simulink model "divergence_sim2"  (R2025b)
settings: Solver=VariableStepAuto  StartTime=0.0  StopTime=3  RelTol=1e-3
PreLoadFcn:
  | % PreLoadFcn - 最小構成
  | stlFile = fullfile(pwd, 'mazeActor.stl');
  | assignin('base', 'stlFile', stlFile);
InitFcn:
  | inputImage = fullfile(pwd, '', 'ex_maze.png');
  | assignin('base', 'mazeInputImage', inputImage);
  | 
  | % InitFcn - 最小構成
  | % Base ワークスペースから変数を取得（無ければエラー）
  | if ~evalin('base','exist(''mazeInputImage'',''var'')')
  |     error('InitFcn:NoInputVar','mazeInputImage not found in base workspace. Ensure PreLoadFcn ran.');
  | end
  | if ~evalin('base','exist(''stlFile'',''var'')')
  |     error('InitFcn:NoSTLVar','stlFile not found in base workspace. Ensure PreLoadFcn ran.');
  | end
  | 
  | inputImage = evalin('base','mazeInputImage');
  | stlFile    = evalin('base','stlFile');
  | 
  | % 入力確認（最小チェック）
  | if ~isfile(inputImage)
  |     error('InitFcn:NoInputFile','Input image not found: %s', inputImage);
  | end
  | 
  | % 実処理：STL 生成（prepareMazeSTL は既存関数と仮定）
  | prepareMazeSTL(inputImage);
  | 
  | % (必要なら prepareMazeSTL 内で stlFile を参照するか、関数に渡す設計にする)
undefined symbols (not defined in the file or in its folder): DiscIntNeverNeededParam, Sim3dSensor
libraries: sim3dlib x3, sim3dgroundtruthsensorlib x3
settings Model: Creator=akina  LastModifiedBy=akina
settings SFSimCC: SimUserSources=cfolder/solver.c  SFSimEcho=off

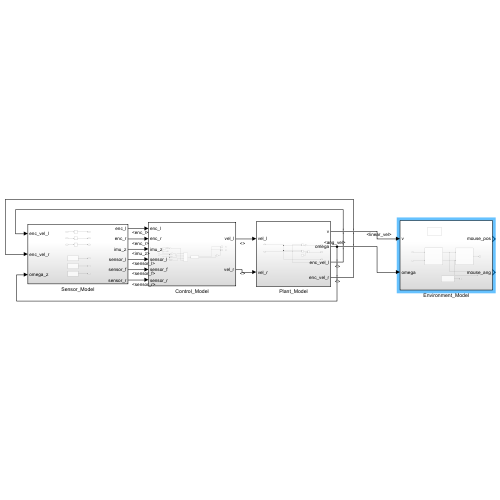
[thumbnail: Simulink's stored preview of the top-level diagram]
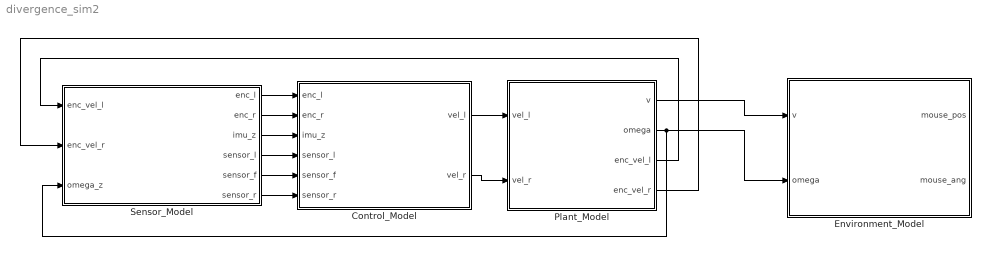
== system divergence_sim2 ==
  Control_Model : Subsystem
  Environment_Model : Subsystem
  Plant_Model : Subsystem
  Sensor_Model : Subsystem
  wires:
  Plant_Model/1(v) -> Environment_Model/1(v)
  Control_Model/1(vel_l) -> Plant_Model/1(vel_l)
  Control_Model/2(vel_r) -> Plant_Model/2(vel_r)
  Plant_Model/2(omega) -> Sensor_Model/3(omega_z), Environment_Model/2(omega)
  Sensor_Model/1(enc_l) -> Control_Model/1(enc_l)
  Sensor_Model/2(enc_r) -> Control_Model/2(enc_r)
  Plant_Model/3(enc_vel_l) -> Sensor_Model/1(enc_vel_l)
  Plant_Model/4(enc_vel_r) -> Sensor_Model/2(enc_vel_r)
  Sensor_Model/3(imu_z) -> Control_Model/3(imu_z)
  Sensor_Model/4(sensor_l) -> Control_Model/4(sensor_l)
  Sensor_Model/5(sensor_f) -> Control_Model/5(sensor_f)
  Sensor_Model/6(sensor_r) -> Control_Model/6(sensor_r)

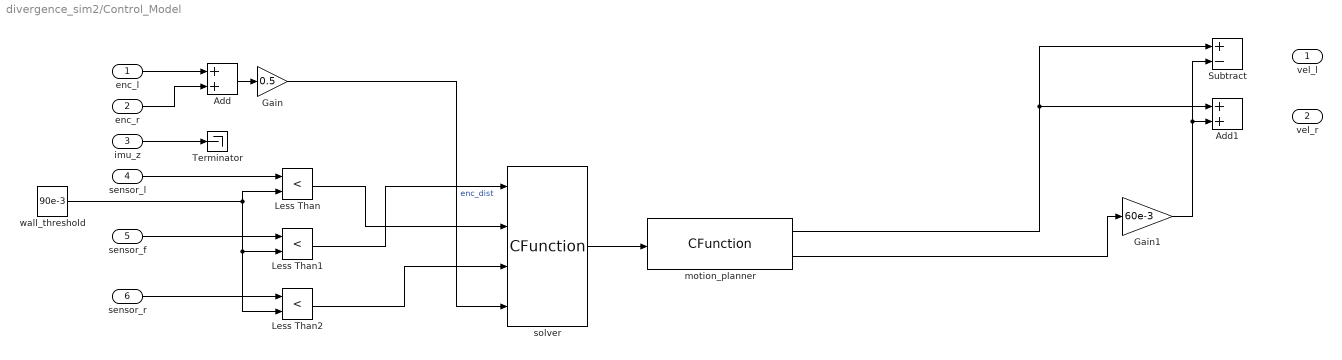
== system divergence_sim2/Control_Model ==
  enc_l : Inport
  enc_r : Inport  Port=2
  imu_z : Inport  Port=3
  sensor_l : Inport  Port=4
  sensor_f : Inport  Port=5
  sensor_r : Inport  Port=6
  Add : Sum
  Add1 : Sum
  Gain : Gain  Gain=0.5
  Gain1 : Gain  Gain=60e-3
  Less Than : RelationalOperator  Operator=<  OutDataTypeStr=boolean  RndMeth=Simplest  InputSameDT=off
  Less Than1 : RelationalOperator  Operator=<  OutDataTypeStr=boolean  RndMeth=Simplest  InputSameDT=off
  Less Than2 : RelationalOperator  Operator=<  OutDataTypeStr=boolean  RndMeth=Simplest  InputSameDT=off
  Subtract : Sum  Inputs=+-
  Terminator : Terminator
  motion_planner : CFunction  OutputCode=|  CodegenOutputCode=|
      OutputCode=|
      | typedef enum {
      |     STOP,
      |     FORWARD,
      |     TURN_LEFT,
      |     TURN_RIGHT,
      |     TURN_BACK
      | } MotionState;
      | 
      | void motion_planner(
      |     int action,
      |     double *v_ref,
      |     double *w_ref)
      | {
      |     static MotionState state = STOP;
      | 
      |     const double V = 0.3;
      |     const double W = 6.0;
      | 
      |     if(action != -1)
      |     {
      |         if(action == 0) state = FORWARD;
      |         if(action == 1) state = TURN_LEFT;
      |         if(action == 2) state = TURN_RIGHT;
      |         if(action == 3) state = TURN_BACK;
      |     }
      | 
      |     switch(state)
      |     {
      |         case FORWARD:
      |             *v_ref = V;
      |             *w_ref = 0;
      |             break;
      | 
      |         case TURN_LEFT:
      |             *v_ref = 0;
      |             *w_ref = W;
      |             break;
      | 
      |         case TURN_RIGHT:
      |             *v_ref = 0;
      |             *w_ref = -W;
      |             break;
      | 
      |         case TURN_BACK:
      |             *v_ref = 0;
      |             *w_ref = W;
      |             break;
      | 
      |         default:
      |             *v_ref = 0;
      |             *w_ref = 0;
      |     }
      | }
      CodegenOutputCode=|
      | typedef enum {
      |     STOP,
      |     FORWARD,
      |     TURN_LEFT,
      |     TURN_RIGHT,
      |     TURN_BACK
      | } MotionState;
      | 
      | void motion_planner(
      |     int action,
      |     double *v_ref,
      |     double *w_ref)
      | {
      |     static MotionState state = STOP;
      | 
      |     const double V = 0.3;
      |     const double W = 6.0;
      | 
      |     if(action != -1)
      |     {
      |         if(action == 0) state = FORWARD;
      |         if(action == 1) state = TURN_LEFT;
      |         if(action == 2) state = TURN_RIGHT;
      |         if(action == 3) state = TURN_BACK;
      |     }
      | 
      |     switch(state)
      |     {
      |         case FORWARD:
      |             *v_ref = V;
      |             *w_ref = 0;
      |             break;
      | 
      |         case TURN_LEFT:
      |             *v_ref = 0;
      |             *w_ref = W;
      |             break;
      | 
      |         case TURN_RIGHT:
      |             *v_ref = 0;
      |             *w_ref = -W;
      |             break;
      | 
      |         case TURN_BACK:
      |             *v_ref = 0;
      |             *w_ref = W;
      |             break;
      | 
      |         default:
      |             *v_ref = 0;
      |             *w_ref = 0;
      |     }
      | }
  solver : CFunction  OutputCode=|  CodegenOutputCode=|
      OutputCode=|
      | void solver(
      |     int front,
      |     int left,
      |     int right,
      |     double distance,
      |     int *action)
      | {
      | 
      |     const double CELL = 0.18;
      |     static double next_call = 0.18;
      | 
      |     *action = -1;
      |     if(distance >= next_cell)
      |     {
      |         if(!left) {
      |         *action = 1;
      |         } else if(!front) {
      |             *action = 0;
      |         } else if(!right) {
      |             *action = 2;
      |         } else {
      |             *action = 3;
      |         }
      |     }
      | }
      CodegenOutputCode=|
      | void solver(
      |     int front,
      |     int left,
      |     int right,
      |     double distance,
      |     int *action)
      | {
      | 
      |     const double CELL = 0.18;
      |     static double next_call = 0.18;
      | 
      |     *action = -1;
      |     if(distance >= next_cell)
      |     {
      |         if(!left) {
      |         *action = 1;
      |         } else if(!front) {
      |             *action = 0;
      |         } else if(!right) {
      |             *action = 2;
      |         } else {
      |             *action = 3;
      |         }
      |     }
      | }
  wall_threshold : Constant  Value=90e-3
  vel_l : Outport
  vel_r : Outport  Port=2
  wires:
  sensor_l/1 -> Less Than/1
  wall_threshold/1 -> Less Than/2, Less Than2/2, Less Than1/2
  sensor_f/1 -> Less Than1/1
  sensor_r/1 -> Less Than2/1
  enc_l/1 -> Add/1
  enc_r/1 -> Add/2
  Add/1 -> Gain/1
  imu_z/1 -> Terminator/1
  motion_planner/2 -> Gain1/1
  Gain1/1 -> Add1/2, Subtract/2
  motion_planner/1 -> Add1/1, Subtract/1
  Less Than/1 -> solver/2
  Less Than1/1 -> solver/1
  Less Than2/1 -> solver/3
  solver/1 -> motion_planner/1
  Gain/1 -> solver/4  "enc_dist"

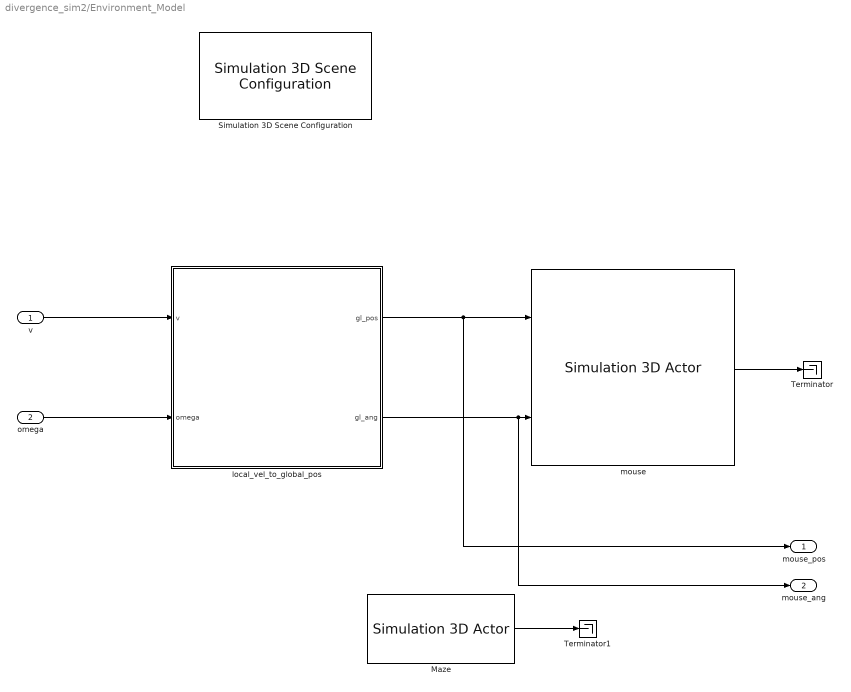
== system divergence_sim2/Environment_Model ==
  v : Inport
  omega : Inport  Port=2
  Maze : sim3dlib/Simulation 3D Actor  Priority=1  ActorName=Sim3dActor1  ParentName=Scene Origin  Operation=Create at setup  InitScriptText=|  SampleTime=-1  Translation=[-0.09 -2.88+0.09 0]  Rotation=[0 0 0]  Scale=[1 1 1]  aMode=5  ActorTag=Sim3dActor1  ActorType=Sim3dActor  ID=1
      | Actor.PreciseContacts = false;
      | Actor.Physics = false;
      | Actor.Color = [1 1 1];
      | actor.Shininess = 0;
      | actor.Metallic = 0;
      | Actor.Collisions = false;
  Simulation 3D Scene Configuration : sim3dlib/Simulation 3D Scene Configuration  Priority=0  ProjectFormat=Default Scenes  SceneDesc=Empty scene  ProjectName=C:\Program Files\MATLAB\R2025b\toolbox\shared\sim3d_projects\automotive_project_windows\UE\WindowsNoEditor\VehicleSimulation.exe  ScenePath=/Game/Maps/HwStrght  EnableOpenDRIVE=off  vehTagList={'Custom';'Scene Origin'}  vehTag=Custom  AttachedCameraRelativeTranslation=[0 0 0]  FreeCameraDefaultInitialTranslation=[-6, 0, 2]  AttachedCameraRelativeRotation=[0 0 0]  FreeCameraDefaultInitialRotation=[0, -15, 0]  ViewpointName=Custom  FreeCameraInitialTranslation=[0 0.6 1.5]  ViewpointTranslation=[0 0 0]  FreeCameraInitialRotation=[0 -90 -90]  ViewpointRotation=[0 0 0]  OpVisEn=off  Ts=.001  EnableWindow=on  EnableRemoteAccess=off  EnableWeather=off  SunAzimuth=90  SunAltitude=40.0  EnableGeospatialSun=off  Latitude=0  Longitude=0  Date=2023-01-01  Time=10:30:00  GeoTimeZone=-5.0  SunDaylightSaving=off  wind=1  clouds=10  EnableVolumetricClouds=off  CloudCoverage=0  CloudAltitude=6  fog=0  rain=0  RaindropsEffect=off  SnowDensity=0  EnableGeospatial=off  TilesetSource=Earth terrain  UseTrueOrigin=off  OriginHeight=200  OriginLatitude=40.744652  OriginLongitude=-73.988864  MapStyle=Aerial  AdditionalAssetIDs=[]  UseAdvancedSunSky=off  SolarTime=11  TimeZone=-5  Day=21  Month=9  Year=2022  UseDaylightSavingTime=on  DSTStartDay=10  DSTStartMonth=3  DSTEndDay=3  DSTEndMonth=11  DSTSwitchHour=2  sensorTag=MainCamera1  sensorId=1  sensorName=MainCamera1  mountLoc=Origin  offsetFlag=off  tmountOffset=[0, 0, 0]  rmountOffset=[0, 0, 0]  HorizontalResolution=1280  VerticalResolution=720  HorizontalFOV=60  mountPoint=[0 0 0]  mountOrientation=[0 0 0]  aMode=5  ID=1  GeoTrigger=Inactive  ViewNameList={'Custom'}  ViewTranslationList={'[0 0.6 1.5]'}  ViewRotationList={'[0 -90 -90]'}
      settings: LibrarySourceBlock=sl3dlib/Simulation 3D/Environment/Simulation 3D Scene Configuration
  Terminator : Terminator
  Terminator1 : Terminator
  local_vel_to_global_pos : Subsystem
  mouse : sim3dlib/Simulation 3D Actor  Priority=1  ActorName=Mouse  ParentName=Scene Origin  Operation=Create at setup  InitScriptText=|  SampleTime=-1  Translation=[0 0 0]  Rotation=[0 0 0]  Scale=[1 1 1]*1e-3  InputsText=Mouse.Translation Mouse.Rotation  aMode=5  ActorTag=Mouse  ActorType=Sim3dActor  ID=C
      | Actor.Shadows = false;
      | Actor.Collisions = false;
      | Actor.Color = [0,0,0];
  mouse_pos : Outport
  mouse_ang : Outport  Port=2
  wires:
  mouse/1 -> Terminator/1
  v/1 -> local_vel_to_global_pos/1(v)
  omega/1 -> local_vel_to_global_pos/2(omega)
  Maze/1 -> Terminator1/1
  local_vel_to_global_pos/1(gl_pos) -> mouse_pos/1, mouse/1
  local_vel_to_global_pos/2(gl_ang) -> mouse_ang/1, mouse/2

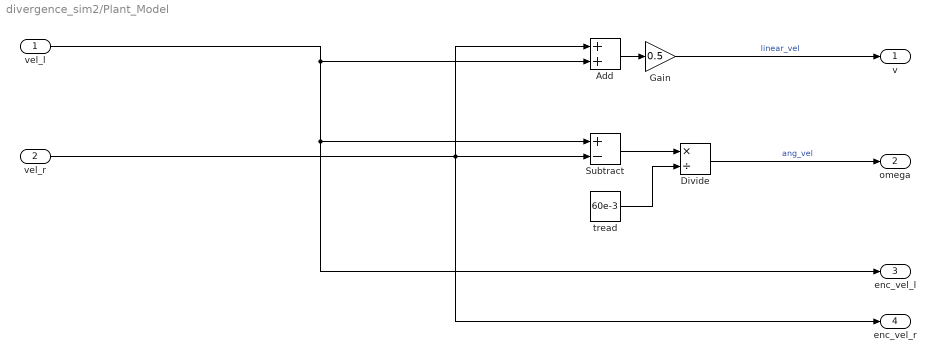
== system divergence_sim2/Plant_Model ==
  vel_l : Inport
  vel_r : Inport  Port=2
  Add : Sum
  Divide : Product  Inputs=*/
  Gain : Gain  Gain=0.5
  Subtract : Sum  Inputs=+-
  tread : Constant  Value=60e-3
  v : Outport
  omega : Outport  Port=2
  enc_vel_l : Outport  Port=3
  enc_vel_r : Outport  Port=4
  wires:
  Add/1 -> Gain/1
  Subtract/1 -> Divide/1
  Divide/1 -> omega/1  "ang_vel"
  tread/1 -> Divide/2
  Gain/1 -> v/1  "linear_vel"
  vel_l/1 -> enc_vel_l/1, Subtract/1, Add/2
  vel_r/1 -> enc_vel_r/1, Subtract/2, Add/1

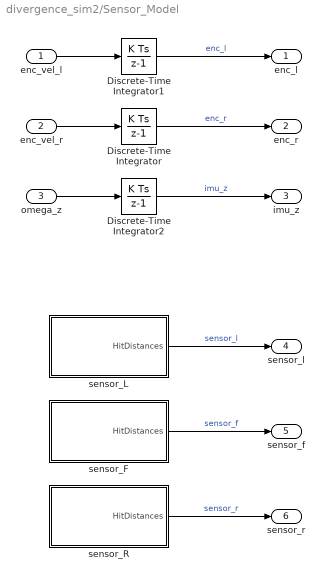
== system divergence_sim2/Sensor_Model ==
  enc_vel_l : Inport
  enc_vel_r : Inport  Port=2
  omega_z : Inport  Port=3
  Discrete-Time Integrator : DiscreteIntegrator  SampleTime=-1  ICPrevOutput=DiscIntNeverNeededParam  ICPrevScaledInput=DiscIntNeverNeededParam
  Discrete-Time Integrator1 : DiscreteIntegrator  SampleTime=-1  ICPrevOutput=DiscIntNeverNeededParam  ICPrevScaledInput=DiscIntNeverNeededParam
  Discrete-Time Integrator2 : DiscreteIntegrator  SampleTime=-1  ICPrevOutput=DiscIntNeverNeededParam  ICPrevScaledInput=DiscIntNeverNeededParam
  sensor_F : Subsystem  mask{pos_x=60, pos_y=0, ang_z=0}
      mask prompts: pos_x "sensor position x (mm)"; pos_y "sensor position y (mm)"; ang_z "sensor rotation z (deg)"
      mask DialogControl ParameterGroupVar Prompt: パラメーター
  sensor_L : Subsystem  mask{pos_x=60, pos_y=0, ang_z=-60}
      mask prompts: pos_x "sensor position x (mm)"; pos_y "sensor position y (mm)"; ang_z "sensor rotation z (deg)"
      mask DialogControl ParameterGroupVar Prompt: パラメーター
  sensor_R : Subsystem  mask{pos_x=60, pos_y=0, ang_z=60}
      mask prompts: pos_x "sensor position x (mm)"; pos_y "sensor position y (mm)"; ang_z "sensor rotation z (deg)"
      mask DialogControl ParameterGroupVar Prompt: パラメーター
  enc_l : Outport
  enc_r : Outport  Port=2
  imu_z : Outport  Port=3
  sensor_l : Outport  Port=4
  sensor_f : Outport  Port=5
  sensor_r : Outport  Port=6
  wires:
  enc_vel_r/1 -> Discrete-Time Integrator/1
  enc_vel_l/1 -> Discrete-Time Integrator1/1
  Discrete-Time Integrator/1 -> enc_r/1  "enc_r"
  Discrete-Time Integrator1/1 -> enc_l/1  "enc_l"
  omega_z/1 -> Discrete-Time Integrator2/1
  Discrete-Time Integrator2/1 -> imu_z/1  "imu_z"
  sensor_F/1(HitDistances) -> sensor_f/1  "sensor_f"
  sensor_R/1(HitDistances) -> sensor_r/1  "sensor_r"
  sensor_L/1(HitDistances) -> sensor_l/1  "sensor_l"

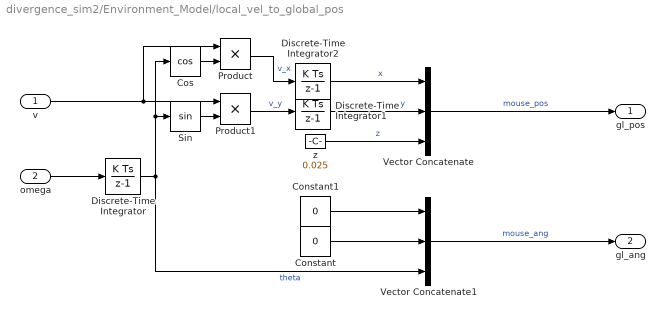
== system divergence_sim2/Environment_Model/local_vel_to_global_pos ==
  v : Inport
  omega : Inport  Port=2
  Constant : Constant  Value=0
  Constant1 : Constant  Value=0
  Cos : Trigonometry  Operator=cos
  Discrete-Time Integrator : DiscreteIntegrator  InitialCondition=-pi/2  SampleTime=-1  ICPrevOutput=DiscIntNeverNeededParam  ICPrevScaledInput=DiscIntNeverNeededParam
  Discrete-Time Integrator1 : DiscreteIntegrator  SampleTime=-1  ICPrevOutput=DiscIntNeverNeededParam  ICPrevScaledInput=DiscIntNeverNeededParam
  Discrete-Time Integrator2 : DiscreteIntegrator  SampleTime=-1  ICPrevOutput=DiscIntNeverNeededParam  ICPrevScaledInput=DiscIntNeverNeededParam
  Product : Product
  Product1 : Product
  Sin : Trigonometry
  Vector Concatenate : Concatenate  NumInputs=3  Mode=Multidimensional array  ConcatenateDimension=2
  Vector Concatenate1 : Concatenate  NumInputs=3  Mode=Multidimensional array  ConcatenateDimension=2
  z : Constant  Value=0.025
  gl_pos : Outport
  gl_ang : Outport  Port=2
  wires:
  omega/1 -> Discrete-Time Integrator/1
  Discrete-Time Integrator/1 -> Vector Concatenate1/3, Sin/1, Cos/1  "theta"
  Product1/1 -> Discrete-Time Integrator1/1  "v_y"
  Product/1 -> Discrete-Time Integrator2/1  "v_x"
  v/1 -> Product1/1, Product/1
  Cos/1 -> Product/2
  Sin/1 -> Product1/2
  Discrete-Time Integrator2/1 -> Vector Concatenate/1  "x"
  Discrete-Time Integrator1/1 -> Vector Concatenate/2  "y"
  z/1 -> Vector Concatenate/3  "z"
  Constant1/1 -> Vector Concatenate1/1
  Constant/1 -> Vector Concatenate1/2
  Vector Concatenate/1 -> gl_pos/1  "mouse_pos"
  Vector Concatenate1/1 -> gl_ang/1  "mouse_ang"

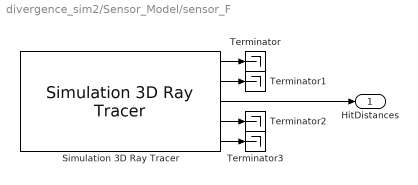
== system divergence_sim2/Sensor_Model/sensor_F ==
  Simulation 3D Ray Tracer : sim3dgroundtruthsensorlib/Simulation 3D Ray Tracer  Priority=1  sensorTag=Sim3dSensor�  sensorId=1  sensorName=Sim3dSensor�  vehTagList={'Mouse';'Scene Origin';'Sim3dActor1'}  vehTag=Mouse  CoordinateSystem=Default  mountLoc=Origin  offsetFlag=on  tmountOffset=[pos_x pos_y 2]  rmountOffset=[0 -pi/2 ang_z/180*pi]  RayOrigins=[0 0 0]  RayDirections=[0 0 1]  RayLengths=4000  NumberOfBounces=0  VisualizeTraceLines=on  EnableOptimization=off  SampleTime=-1  mountPoint=[60 0 2]  mountOrientation=[0 -1.5707963267949 0]  aMode=5  ID=1
      settings: LibrarySourceBlock=sl3dlib/Simulation 3D/Sensors/Simulation 3D Ray Tracer
  Terminator{,1..3} (4 alike) : Terminator
  HitDistances : Outport
  wires:
  Simulation 3D Ray Tracer/3 -> HitDistances/1
  Simulation 3D Ray Tracer/2 -> Terminator1/1
  Simulation 3D Ray Tracer/4 -> Terminator2/1
  Simulation 3D Ray Tracer/5 -> Terminator3/1
  Simulation 3D Ray Tracer/1 -> Terminator/1

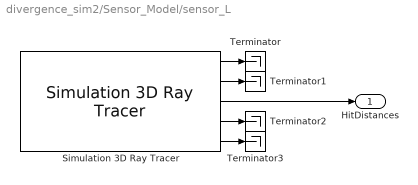
== system divergence_sim2/Sensor_Model/sensor_L ==
  Simulation 3D Ray Tracer : sim3dgroundtruthsensorlib/Simulation 3D Ray Tracer  Priority=1  sensorTag=Sim3dSensor�  sensorId=3  sensorName=Sim3dSensor�  vehTagList={'Mouse';'Scene Origin';'Sim3dActor1'}  vehTag=Mouse  CoordinateSystem=Default  mountLoc=Origin  offsetFlag=on  tmountOffset=[pos_x pos_y 2]  rmountOffset=[0 -pi/2 ang_z/180*pi]  RayOrigins=[0 0 0]  RayDirections=[0 0 1]  RayLengths=4000  NumberOfBounces=0  VisualizeTraceLines=on  EnableOptimization=off  SampleTime=-1  mountPoint=[60 0 2]  mountOrientation=[0 -1.5707963267949 -1.0471975511966]  aMode=5  ID=3
      settings: LibrarySourceBlock=sl3dlib/Simulation 3D/Sensors/Simulation 3D Ray Tracer
  Terminator{,1..3} (4 alike) : Terminator
  HitDistances : Outport
  wires:
  Simulation 3D Ray Tracer/3 -> HitDistances/1
  Simulation 3D Ray Tracer/2 -> Terminator1/1
  Simulation 3D Ray Tracer/4 -> Terminator2/1
  Simulation 3D Ray Tracer/5 -> Terminator3/1
  Simulation 3D Ray Tracer/1 -> Terminator/1

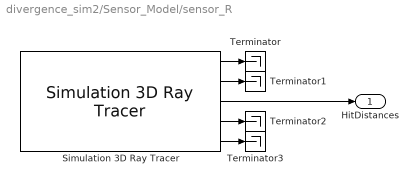
== system divergence_sim2/Sensor_Model/sensor_R ==
  Simulation 3D Ray Tracer : sim3dgroundtruthsensorlib/Simulation 3D Ray Tracer  Priority=1  sensorTag=Sim3dSensor�  sensorId=2  sensorName=Sim3dSensor�  vehTagList={'Mouse';'Scene Origin';'Sim3dActor1'}  vehTag=Mouse  CoordinateSystem=Default  mountLoc=Origin  offsetFlag=on  tmountOffset=[pos_x pos_y 2]  rmountOffset=[0 -pi/2 ang_z/180*pi]  RayOrigins=[0 0 0]  RayDirections=[0 0 1]  RayLengths=4000  NumberOfBounces=0  VisualizeTraceLines=on  EnableOptimization=off  SampleTime=-1  mountPoint=[60 0 2]  mountOrientation=[0 -1.5707963267949 1.0471975511966]  aMode=5  ID=2
      settings: LibrarySourceBlock=sl3dlib/Simulation 3D/Sensors/Simulation 3D Ray Tracer
  Terminator{,1..3} (4 alike) : Terminator
  HitDistances : Outport
  wires:
  Simulation 3D Ray Tracer/3 -> HitDistances/1
  Simulation 3D Ray Tracer/2 -> Terminator1/1
  Simulation 3D Ray Tracer/4 -> Terminator2/1
  Simulation 3D Ray Tracer/5 -> Terminator3/1
  Simulation 3D Ray Tracer/1 -> Terminator/1
